simulink model "Ch2CSTRClosedLoop_Sys"  (R2020a)
settings: Solver=ode45  StartTime=0.0  StopTime=10.0  RelTol=1e-5  EnableMultiTasking=on
values from neighbouring files (symbols this model uses):
  alpha = 0.1    [Ch2CSTRClosedLoop.m]    (also in Ch2CSTRClosedLoopRobustness.m)
  beta = 0.5    [Ch2CSTRClosedLoop.m]    (also in Ch2CSTRClosedLoopRobustness.m = 0)
  C_Afeed = 10    [Ch2CSTRClosedLoop.m]    (also in Ch2CSTRClosedLoopRobustness.m; Ch2CSTROpenLoop.m)
  C_Afeed_Change = 5    [Ch2CSTRClosedLoop.m]    (also in Ch2CSTRClosedLoopRobustness.m = 10; Ch2CSTROpenLoop.m = -10)
  C_Afeed_instant = 2    [Ch2CSTRClosedLoop.m]    (also in Ch2CSTRClosedLoopRobustness.m; Ch2CSTROpenLoop.m = 10)
  C_Bin = 70    [Ch2CSTRClosedLoop.m]    (also in Ch2CSTRClosedLoopRobustness.m)
  CB_Change = 5    [Ch2CSTRClosedLoop.m]    (also in Ch2CSTRClosedLoopRobustness.m = 0)
  CB_instant = 20    [Ch2CSTRClosedLoop.m]    (also in Ch2CSTRClosedLoopRobustness.m = 10)
  Fr_Change = 5    [Ch2CSTRClosedLoop.m]    (also in Ch2CSTRClosedLoopRobustness.m = 0; Ch2CSTROpenLoop.m = 20)
  Fr_in = 60    [Ch2CSTRClosedLoop.m]    (also in Ch2CSTRClosedLoopRobustness.m; Ch2CSTROpenLoop.m)
  Fr_instant = 10    [Ch2CSTRClosedLoop.m]    (also in Ch2CSTRClosedLoopRobustness.m = 2; Ch2CSTROpenLoop.m = 2)
  gamma = 0    [Ch2CSTRClosedLoop.m]    (also in Ch2CSTRClosedLoopRobustness.m)
  Kp = 3.33    [Ch2CSTRClosedLoop.m]    (also in Ch2CSTRClosedLoopRobustness.m = 2.372)
  Ref_C_B_Change = 0    [Ch2CSTRClosedLoop.m]    (also in Ch2CSTRClosedLoopRobustness.m)
  Ref_C_B_instant = 2    [Ch2CSTRClosedLoop.m]    (also in Ch2CSTRClosedLoopRobustness.m)
  Td = 0.18    [Ch2CSTRClosedLoop.m]    (also in Ch2CSTRClosedLoopRobustness.m = 0.162)
  Ti = 0.685    [Ch2CSTRClosedLoop.m]    (also in Ch2CSTRClosedLoopRobustness.m = 0.663)
settings Model: Creator=rvilanova  LastModifiedBy=rvilanova
settings DataIOCC: LimitDataPoints=on  SaveFormat=Array  ReturnWorkspaceOutputs=off
settings OptimizationCC: LifeSpan=inf
settings DebuggingCC: SFUnexpectedBacktrackingDiag=warning  SFNoUnconditionalDefaultTransitionDiag=warning  SFExecutionAtInitializationDiag=none  ArithmeticOperatorsInVariantConditions=warning
settings HardwareCC: ProdBitPerPointer=32  ProdBitPerSizeT=32  ProdBitPerPtrDiffT=32  ProdLargestAtomicFloat=None  ProdIntDivRoundTo=Undefined  ProdEndianess=Unspecified  ProdWordSize=32  ProdHWDeviceType=32-bit Generic
settings ModelReferenceCC: PropagateSignalLabelsOutOfModel=off
settings SFSimCC: SimUseLocalCustomCode=off  CustomCodeUndefinedFunction=UseInterfaceOnly
settings RTWCC: RTWUseLocalCustomCode=off
settings CodeAppCC: StateflowObjectComments=on
settings GRTTargetCC: TargetLangStandard=C89/C90 (ANSI)
settings ConfigComp: CovMetricSettings=dw  CovHtmlReporting=on  CovSaveCumulativeToWorkspaceVar=on  CovSaveSingleToWorkspaceVar=on  CovExternalEMLEnable=off  CovSFcnEnable=off

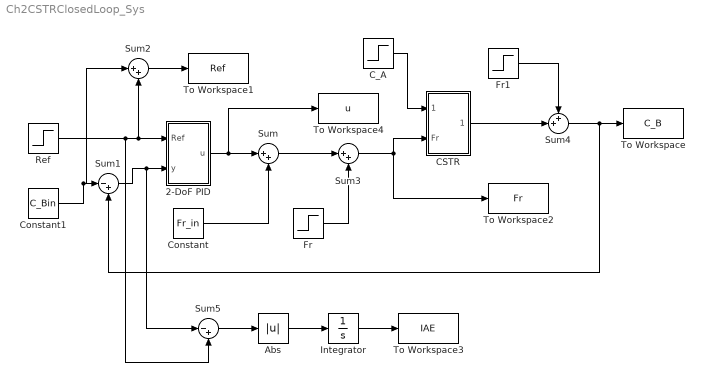
== system Ch2CSTRClosedLoop_Sys ==
  2-DoF PID : Subsystem
  Abs : Abs
  "CSTR " : Subsystem
  C_A : Step  Time=C_Afeed_instant  Before=C_Afeed  After=C_Afeed*(1+C_Afeed_Change/100)  SampleTime=0
  Constant : Constant  Value=Fr_in
  Constant1 : Constant  Value=C_Bin
  Fr : Step  Time=Fr_instant  After=Fr_Change  SampleTime=0
  Fr1 : Step  Time=CB_instant  After=CB_Change  SampleTime=0
  Integrator : Integrator
  Ref : Step  Time=Ref_C_B_instant  After=Ref_C_B_Change
  Sum : Sum  Inputs=|++
  Sum1 : Sum  Inputs=|-+
  Sum2 : Sum  Inputs=|++
  Sum3 : Sum  Inputs=|++
  Sum4 : Sum  Inputs=++|
  Sum5 : Sum  Inputs=|-+
  To Workspace : ToWorkspace  VariableName=C_B  SaveFormat=Timeseries  SampleTime=-1
  To Workspace1 : ToWorkspace  VariableName=Ref  SaveFormat=Timeseries  SampleTime=-1
  To Workspace2 : ToWorkspace  VariableName=Fr  SaveFormat=Timeseries  SampleTime=-1
  To Workspace3 : ToWorkspace  VariableName=IAE  SaveFormat=Timeseries  SampleTime=-1
  To Workspace4 : ToWorkspace  VariableName=u  SaveFormat=Timeseries  SampleTime=1
  wires:
  C_A/1 -> "CSTR "/1(C_A)
  Constant/1 -> Sum/2
  Ref/1 -> Sum5/2, Sum2/2, 2-DoF PID/1(Ref)
  Sum1/1 -> Sum5/1, 2-DoF PID/2(y)
  2-DoF PID/1(u) -> To Workspace4/1, Sum/1
  Constant1/1 -> Sum2/1, Sum1/1
  Sum2/1 -> To Workspace1/1
  Sum/1 -> Sum3/1
  Sum3/1 -> To Workspace2/1, "CSTR "/2(Fr)
  Fr/1 -> Sum3/2
  "CSTR "/1(C_B) -> Sum4/2
  Fr1/1 -> Sum4/1
  Sum4/1 -> Sum1/2, To Workspace/1
  Sum5/1 -> Abs/1
  Abs/1 -> Integrator/1
  Integrator/1 -> To Workspace3/1

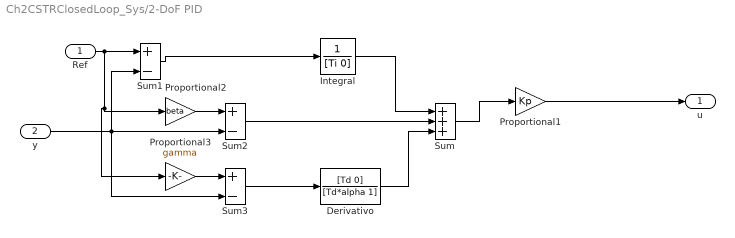
== system Ch2CSTRClosedLoop_Sys/2-DoF PID ==
  Ref : Inport
  y : Inport  Port=2
  Derivativo : TransferFcn  Numerator=[Td 0]  Denominator=[Td*alpha 1]
  Integral : TransferFcn  Denominator=[Ti 0]
  Proportional1 : Gain  Gain=Kp  SaturateOnIntegerOverflow=on  OutDataTypeStr=Inherit: Same as input  ParamDataTypeStr=Inherit: Same as input
  Proportional2 : Gain  Gain=beta  SaturateOnIntegerOverflow=on  OutDataTypeStr=Inherit: Same as input  ParamDataTypeStr=Inherit: Same as input
  Proportional3 : Gain  Gain=gamma  SaturateOnIntegerOverflow=on  OutDataTypeStr=Inherit: Same as input  ParamDataTypeStr=Inherit: Same as input
  Sum : Sum  Inputs=+++  InputSameDT=on  SaturateOnIntegerOverflow=on  OutDataTypeStr=Inherit: Same as first input
  Sum1 : Sum  Inputs=+-  InputSameDT=on  SaturateOnIntegerOverflow=on  OutDataTypeStr=Inherit: Same as first input
  Sum2 : Sum  Inputs=+-  InputSameDT=on  SaturateOnIntegerOverflow=on  OutDataTypeStr=Inherit: Same as first input
  Sum3 : Sum  Inputs=+-  InputSameDT=on  SaturateOnIntegerOverflow=on  OutDataTypeStr=Inherit: Same as first input
  u : Outport
  wires:
  Sum1/1 -> Integral/1
  y/1 -> Sum1/2, Sum3/2, Sum2/2
  Sum/1 -> Proportional1/1
  Sum3/1 -> Derivativo/1
  Integral/1 -> Sum/1
  Sum2/1 -> Sum/2
  Proportional2/1 -> Sum2/1
  Proportional3/1 -> Sum3/1
  Ref/1 -> Proportional3/1, Proportional2/1, Sum1/1
  Derivativo/1 -> Sum/3
  Proportional1/1 -> u/1

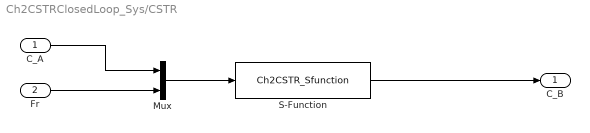
== system Ch2CSTRClosedLoop_Sys/CSTR  ==
  C_A : Inport
  Fr : Inport  Port=2
  Mux : Mux  Inputs=2
  S-Function : S-Function  FunctionName=Ch2CSTR_Sfunction  Parameters=C_Ao, C_Bo  SFunctionDeploymentMode=off  EnableBusSupport=off
  C_B : Outport
  wires:
  S-Function/1 -> C_B/1
  Mux/1 -> S-Function/1
  Fr/1 -> Mux/2
  C_A/1 -> Mux/1
